simulink model "SwLegComp"  (R2015a)
settings: Solver=ode45  StartTime=0.0  StopTime=10.0  RelTol=1e-3
settings Model: Creator=smsong  LastModifiedBy=smsong

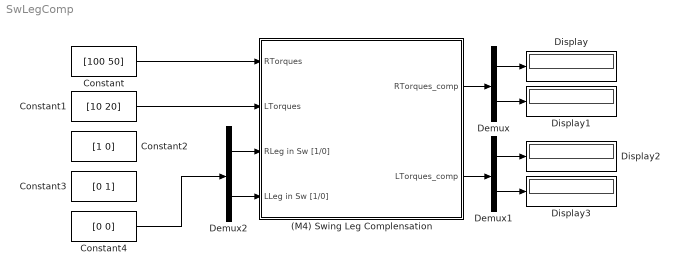
== system SwLegComp ==
  (M4) Swing Leg Complensation : Subsystem
  Constant : Constant  Value=[100 50]
  Constant1 : Constant  Value=[10 20]
  Constant2 : Constant  Value=[1 0]
  Constant3 : Constant  Value=[0 1]
  Constant4 : Constant  Value=[0 0]
  Demux : Demux  Outputs=2
  Demux1 : Demux  Outputs=2
  Demux2 : Demux  Outputs=2
  Display{,1..3} (4 alike) : Display
  wires:
  Constant/1 -> (M4) Swing Leg Complensation/1(RTorques)
  Constant1/1 -> (M4) Swing Leg Complensation/2(LTorques)
  (M4) Swing Leg Complensation/1(RTorques_comp) -> Demux/1
  Demux/1 -> Display/1
  Demux/2 -> Display1/1
  (M4) Swing Leg Complensation/2(LTorques_comp) -> Demux1/1
  Demux1/1 -> Display2/1
  Demux1/2 -> Display3/1
  Demux2/1 -> (M4) Swing Leg Complensation/3(RLeg in Sw [1/0])
  Demux2/2 -> (M4) Swing Leg Complensation/4(LLeg in Sw [1/0])
  Constant4/1 -> Demux2/1

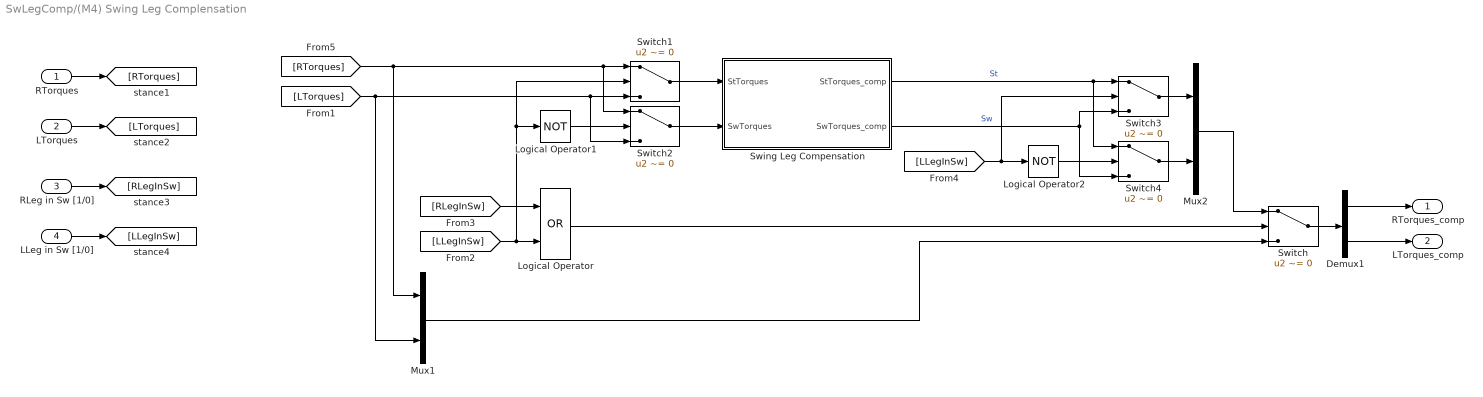
== system SwLegComp/(M4) Swing Leg Complensation ==
  RTorques : Inport
  LTorques : Inport  Port=2
  RLeg in Sw [1/0] : Inport  Port=3
  LLeg in Sw [1/0] : Inport  Port=4
  Demux1 : Demux  Outputs=2
  Logical Operator : Logic  Operator=OR  AllPortsSameDT=off  OutDataTypeStr=boolean
  Logical Operator1 : Logic  Operator=NOT  AllPortsSameDT=off  OutDataTypeStr=boolean
  Logical Operator2 : Logic  Operator=NOT  AllPortsSameDT=off  OutDataTypeStr=boolean
  Mux1 : Mux  Inputs=2
  Mux2 : Mux  Inputs=2
  Swing Leg Compensation : Subsystem
  Switch{,1..4} (5 alike) : Switch  Criteria=u2 ~= 0
  RTorques_comp : Outport
  LTorques_comp : Outport  Port=2
  wires:
  [LLegInSw] -> Logical Operator1/1, Switch1/2, Logical Operator/2
  [RLegInSw] -> Logical Operator/1
  Logical Operator/1 -> Switch/2
  [LTorques] -> Mux1/2, Switch2/3, Switch1/3
  [RTorques] -> Switch2/1, Switch1/1, Mux1/1
  Switch1/1 -> Swing Leg Compensation/1(StTorques)
  Logical Operator1/1 -> Switch2/2
  Switch2/1 -> Swing Leg Compensation/2(SwTorques)
  Swing Leg Compensation/1(StTorques_comp) -> Switch4/1, Switch3/1  "St"
  Swing Leg Compensation/2(SwTorques_comp) -> Switch3/3, Switch4/3  "Sw"
  RTorques/1 -> [RTorques]
  LTorques/1 -> [LTorques]
  RLeg in Sw [1/0]/1 -> [RLegInSw]
  LLeg in Sw [1/0]/1 -> [LLegInSw]
  [LLegInSw] -> Logical Operator2/1, Switch3/2
  Logical Operator2/1 -> Switch4/2
  Switch3/1 -> Mux2/1
  Switch4/1 -> Mux2/2
  Mux2/1 -> Switch/1
  Mux1/1 -> Switch/3
  Switch/1 -> Demux1/1
  Demux1/1 -> RTorques_comp/1
  Demux1/2 -> LTorques_comp/1

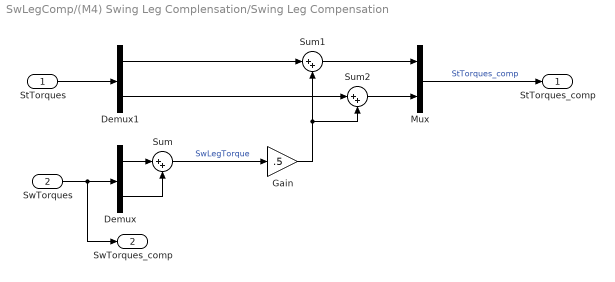
== system SwLegComp/(M4) Swing Leg Complensation/Swing Leg Compensation ==
  StTorques : Inport
  SwTorques : Inport  Port=2
  Demux : Demux  Outputs=2
  Demux1 : Demux  Outputs=2
  Gain : Gain  Gain=.5
  Mux : Mux  Inputs=2
  Sum : Sum  Inputs=|++
  Sum1 : Sum  Inputs=|++
  Sum2 : Sum  Inputs=|++
  StTorques_comp : Outport
  SwTorques_comp : Outport  Port=2
  wires:
  Demux1/1 -> Sum1/1
  Sum/1 -> Gain/1  "SwLegTorque"
  Demux/1 -> Sum/1
  Demux1/2 -> Sum2/1
  Demux/2 -> Sum/2
  StTorques/1 -> Demux1/1
  Mux/1 -> StTorques_comp/1  "StTorques_comp"
  SwTorques/1 -> Demux/1, SwTorques_comp/1
  Sum2/1 -> Mux/2
  Gain/1 -> Sum1/2, Sum2/2
  Sum1/1 -> Mux/1
